simulink model "Tangentialkraftverteilung"  (R2019b)
settings: Solver=VariableStepAuto  StartTime=0.0  StopTime=10.0  RelTol=1e-3
model workspace (MAT data in the model file):
  h_s = 0.5
  l = 2.8
  l_v = 1.344
settings Model: OrderedModelArguments=off  Creator=lenan  LastModifiedBy=lenan

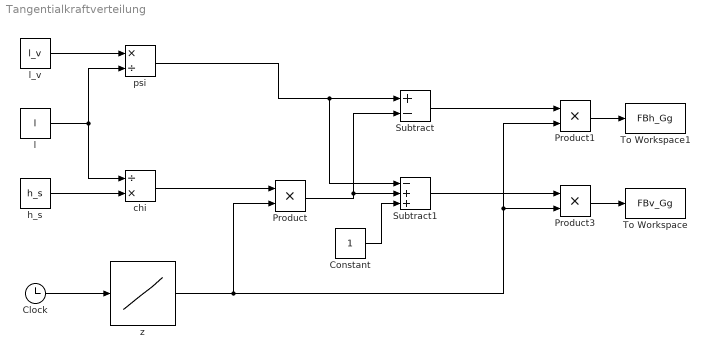
== system Tangentialkraftverteilung ==
  Clock : Clock
  Constant : Constant
  Product : Product
  Product1 : Product
  Product3 : Product
  Subtract : Sum  Inputs=+-
  Subtract1 : Sum  Inputs=-++
  To Workspace : ToWorkspace  VariableName=FBv_Gg  SaveFormat=Timeseries  SampleTime=-1
  To Workspace1 : ToWorkspace  VariableName=FBh_Gg  SaveFormat=Timeseries  SampleTime=-1
  chi : Product  Inputs=/*
  h_s : Constant  Value=h_s
  l : Constant  Value=l
  l_v : Constant  Value=l_v
  psi : Product  Inputs=*/
  z : Lookup_n-D  NumberOfTableDimensions=1  BreakpointsForDimension1=[0.01 ((l_v/l)/(h_s/l))-(-(1-l_v/l)/(h_s/l))]  Table=[(-(1-l_v/l)/(h_s/l)) ((l_v/l)/(h_s/l))]  InternalRulePriority=Speed  RndMeth=Simplest  InputSameDT=on
  wires:
  l_v/1 -> psi/1
  l/1 -> chi/1, psi/2
  h_s/1 -> chi/2
  Clock/1 -> z/1
  z/1 -> Product/2, Product3/2, Product1/2
  chi/1 -> Product/1
  psi/1 -> Subtract1/1, Subtract/1
  Subtract/1 -> Product1/1
  Product/1 -> Subtract1/2, Subtract/2
  Constant/1 -> Subtract1/3
  Subtract1/1 -> Product3/1
  Product1/1 -> To Workspace1/1
  Product3/1 -> To Workspace/1
